simulink model "LS_MRAC"  (Simulink 10.3)
settings: Solver=ode45  StartTime=10  StopTime=20  RelTol=1e-3  AbsTol=1e-6
values from neighbouring files (symbols this model uses):
  Af = zeros(nf); Af(1:nf-1, 2:nf) = eye(nf-1); Af(end, :) = -fliplr(den(2:end))    [LS_MRAC_sim.m]
  Bf = zeros(nf,1); Bf(end) = 1    [LS_MRAC_sim.m]
  DC = 3    [LS_MRAC_sim.m]
  gamma = 20    [LS_MRAC_sim.m]
  kp = 1/3    (= 0.333333333333)    [LS_MRAC_sim.m]    (also in controle2DOF.m = N_p(find(N_p ~= 0, 1, 'first')))
  l0 = 2    [LS_MRAC_sim.m]
  R0 = 20*eye(2*n)    [LS_MRAC_sim.m]
  st = 0.01    [LS_MRAC_sim.m]
  theta0 = zeros(2*n, 1)    [LS_MRAC_sim.m]
libraries: cstblocks x2
settings Model: LogicAnalyzerSignalOrdering=8b4a3e7d-a8a8-4c3d-8b08-fef628b084f5,c1fd59b2-397d-4e52-bac2-f1ea190e9af4,0804b0ab-6626-4093-842a-42967a9eb430  Creator=Ramon  LastModifiedBy=Lucas  MultithreadedSim=on
settings SolverCC: AutoScaleAbsTol=off
settings DataIOCC: SaveOutput=off  SaveTime=off
settings OptimizationCC: BlockReduction=off  BooleanDataType=off  InitFltsAndDblsToZero=on
settings DebuggingCC: SaveWithParameterizedLinksMsg=none  SignalResolutionControl=TryResolveAllWithWarning  MultiTaskDSMMsg=warning  MultiTaskCondExecSysMsg=none
settings HardwareCC: TargetUnknown=on
settings RTWCC: TemplateMakefile=grt_vc.tmf

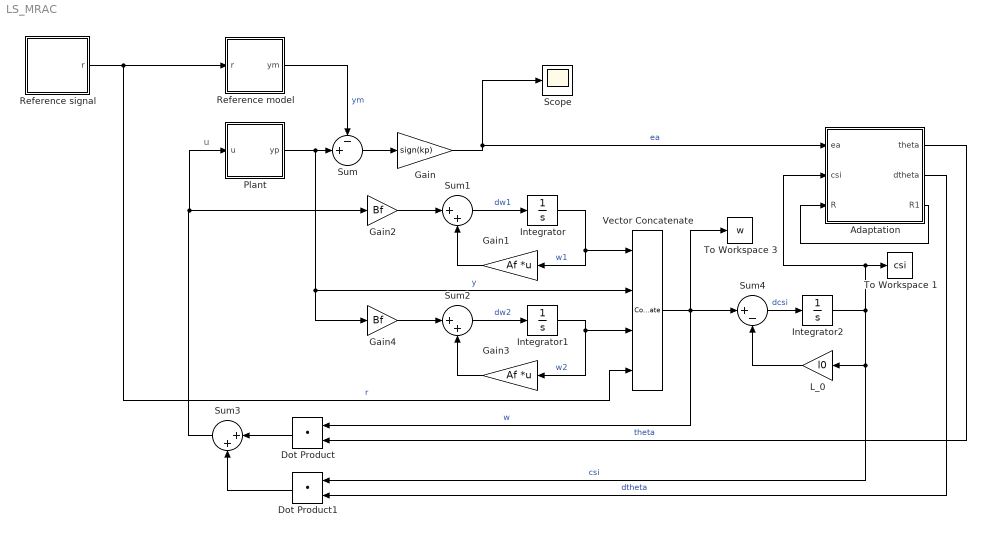
== system LS_MRAC ==
  note: u
  Adaptation : Subsystem
  Dot Product : DotProduct  InputSameDT=on  OutDataTypeStr=Inherit: Inherit via internal rule
  Dot Product1 : DotProduct  InputSameDT=on  OutDataTypeStr=Inherit: Inherit via internal rule
  Gain : Gain  Gain=sign(kp)
  Gain1 : Gain  Gain=Af  Multiplication=Matrix(K*u) (u vector)
  Gain2 : Gain  Gain=Bf
  Gain3 : Gain  Gain=Af  Multiplication=Matrix(K*u) (u vector)
  Gain4 : Gain  Gain=Bf
  Integrator : Integrator
  Integrator1 : Integrator
  Integrator2 : Integrator
  L_0 : Gain  Gain=l0
  Plant : Subsystem
  Reference model : Subsystem
  Reference signal : Subsystem
  Scope : Scope
  Sum : Sum  Inputs=-+|  InputSameDT=on  SaturateOnIntegerOverflow=on  OutDataTypeStr=Inherit: Same as first input
  Sum1 : Sum  Inputs=|++  InputSameDT=on  SaturateOnIntegerOverflow=on  OutDataTypeStr=Inherit: Same as first input
  Sum2 : Sum  Inputs=|++  InputSameDT=on  SaturateOnIntegerOverflow=on  OutDataTypeStr=Inherit: Same as first input
  Sum3 : Sum  Inputs=|++  InputSameDT=on  SaturateOnIntegerOverflow=on  OutDataTypeStr=Inherit: Same as first input
  Sum4 : Sum  Inputs=|+-  InputSameDT=on  SaturateOnIntegerOverflow=on  OutDataTypeStr=Inherit: Same as first input
  To Workspace 1 : ToWorkspace  VariableName=csi  SampleTime=st
  To Workspace 3 : ToWorkspace  VariableName=w  SampleTime=st
  Vector Concatenate : Concatenate  NumInputs=4
  wires:
  Reference model/1(ym) -> Sum/1  "ym"
  Plant/1(yp) -> Gain4/1, Vector Concatenate/2, Sum/2  "y"
  Sum3/1 -> Plant/1(u), Gain2/1
  Adaptation/1(theta) -> Dot Product/2  "theta"
  Gain/1 -> Scope/1, Adaptation/1(ea)  "ea"
  Sum/1 -> Gain/1
  Sum1/1 -> Integrator/1  "dw1"
  Gain2/1 -> Sum1/1
  Integrator/1 -> Vector Concatenate/1, Gain1/1  "w1"
  Gain1/1 -> Sum1/2
  Sum2/1 -> Integrator1/1  "dw2"
  Reference signal/1(r) -> Vector Concatenate/4, Reference model/1(r)  "r"
  Integrator1/1 -> Gain3/1, Vector Concatenate/3  "w2"
  Gain3/1 -> Sum2/2
  Gain4/1 -> Sum2/1
  Vector Concatenate/1 -> Dot Product/1, To Workspace 3/1, Sum4/1  "w"
  Integrator2/1 -> To Workspace 1/1, Adaptation/2(csi), L_0/1, Dot Product1/1  "csi"
  Dot Product/1 -> Sum3/1
  Dot Product1/1 -> Sum3/2
  Adaptation/2(dtheta) -> Dot Product1/2  "dtheta"
  Sum4/1 -> Integrator2/1  "dcsi"
  L_0/1 -> Sum4/2
  Adaptation/3(R1) -> Adaptation/3(R)

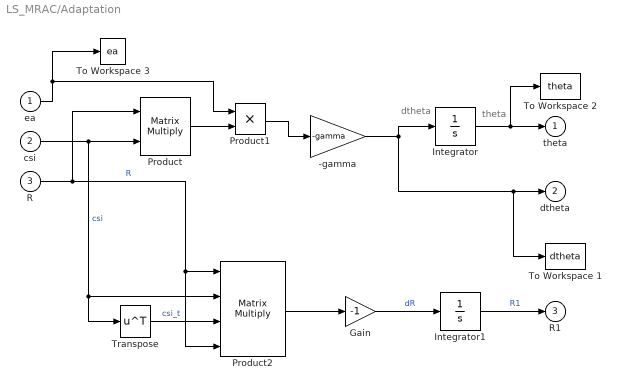
== system LS_MRAC/Adaptation ==
  note: theta
  note: dtheta
  ea : Inport  PortDimensions=1
  csi : Inport  Port=2
  R : Inport  Port=3
  -gamma : Gain  Gain=-gamma  SaturateOnIntegerOverflow=on  OutDataTypeStr=Inherit: Same as input  ParamDataTypeStr=Inherit: Same as input
  Gain : Gain  Gain=-1
  Integrator : Integrator  InitialCondition=theta0
  Integrator1 : Integrator  InitialCondition=R0
  Product : Product  Multiplication=Matrix(*)  InputSameDT=on  RndMeth=Zero  SaturateOnIntegerOverflow=on  OutDataTypeStr=Inherit: Same as first input
  Product1 : Product
  Product2 : Product  Inputs=4  Multiplication=Matrix(*)  InputSameDT=on  RndMeth=Zero  SaturateOnIntegerOverflow=on  OutDataTypeStr=Inherit: Same as first input
  To Workspace 1 : ToWorkspace  VariableName=dtheta  SampleTime=st
  To Workspace 2 : ToWorkspace  VariableName=theta  SampleTime=st
  To Workspace 3 : ToWorkspace  VariableName=ea  SampleTime=st
  Transpose : Math  Operator=transpose  SaturateOnIntegerOverflow=on
  theta : Outport  InitialOutput=0  VectorParamsAs1DForOutWhenUnconnected=off
  dtheta : Outport  Port=2  InitialOutput=0  VectorParamsAs1DForOutWhenUnconnected=off
  R1 : Outport  Port=3  InitialOutput=0  VectorParamsAs1DForOutWhenUnconnected=off
  wires:
  Integrator/1 -> To Workspace 2/1, theta/1
  -gamma/1 -> Integrator/1, To Workspace 1/1, dtheta/1
  ea/1 -> Product1/1, To Workspace 3/1
  Integrator1/1 -> R1/1  "R1"
  Product2/1 -> Gain/1
  Transpose/1 -> Product2/3  "csi_t"
  Product/1 -> Product1/2
  csi/1 -> Product/2, Transpose/1, Product2/2  "csi"
  R/1 -> Product/1, Product2/4, Product2/1  "R"
  Gain/1 -> Integrator1/1  "dR"
  Product1/1 -> -gamma/1

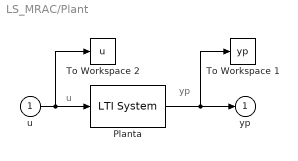
== system LS_MRAC/Plant ==
  note: yp
  note: u
  u : Inport
  Planta : cstblocks/LTI System  sys=P  IC=x0
  To Workspace 1 : ToWorkspace  VariableName=yp  SampleTime=st
  To Workspace 2 : ToWorkspace  VariableName=u  SampleTime=st
  yp : Outport  InitialOutput=0  VectorParamsAs1DForOutWhenUnconnected=off
  wires:
  u/1 -> To Workspace 2/1, Planta/1
  Planta/1 -> yp/1, To Workspace 1/1

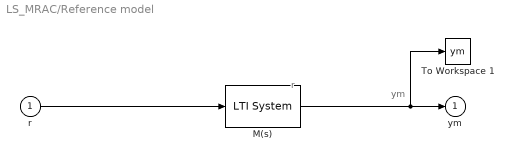
== system LS_MRAC/Reference model ==
  note: r
  note: ym
  r : Inport
  M(s) : cstblocks/LTI System  sys=M  IC=xm0
  To Workspace 1 : ToWorkspace  VariableName=ym  SampleTime=st
  ym : Outport  InitialOutput=0  VectorParamsAs1DForOutWhenUnconnected=off
  wires:
  M(s)/1 -> To Workspace 1/1, ym/1
  r/1 -> M(s)/1

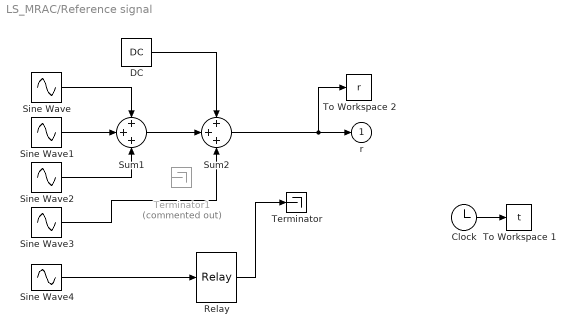
== system LS_MRAC/Reference signal ==
  Clock : Clock
  DC : Constant  Value=DC
  Relay : Relay  OnOutputValue=10  OffOutputValue=-10
  Sine Wave : Sin  SampleTime=0
  Sine Wave1 : Sin  Frequency=3  SampleTime=0
  Sine Wave2 : Sin  Frequency=5  SampleTime=0
  Sine Wave3 : Sin  Frequency=7  SampleTime=0
  Sine Wave4 : Sin  Frequency=0.1*pi  SampleTime=0
  Sum1 : Sum  Inputs=+++  InputSameDT=on  SaturateOnIntegerOverflow=on  OutDataTypeStr=Inherit: Same as first input
  Sum2 : Sum  Inputs=+++  InputSameDT=on  SaturateOnIntegerOverflow=on  OutDataTypeStr=Inherit: Same as first input
  Terminator : Terminator
  Terminator1 : Terminator  Commented=on
  To Workspace 1 : ToWorkspace  VariableName=t  SampleTime=st
  To Workspace 2 : ToWorkspace  VariableName=r  SampleTime=st
  r : Outport  InitialOutput=0  VectorParamsAs1DForOutWhenUnconnected=off
  wires:
  DC/1 -> Sum2/1
  Sum2/1 -> To Workspace 2/1, r/1
  Clock/1 -> To Workspace 1/1
  Sine Wave1/1 -> Sum1/2
  Sine Wave/1 -> Sum1/1
  Sine Wave2/1 -> Sum1/3
  Sine Wave3/1 -> Sum2/3
  Sum1/1 -> Sum2/2
  Sine Wave4/1 -> Relay/1
  Relay/1 -> Terminator/1
